simulink model "Simulacion_Realimentacion_del_estado"  (R2017b)
settings: Solver=VariableStepAuto  StartTime=0.0  StopTime=540  RelTol=1e-3
settings Model: Creator=CPOH  LastModifiedBy=CPOH

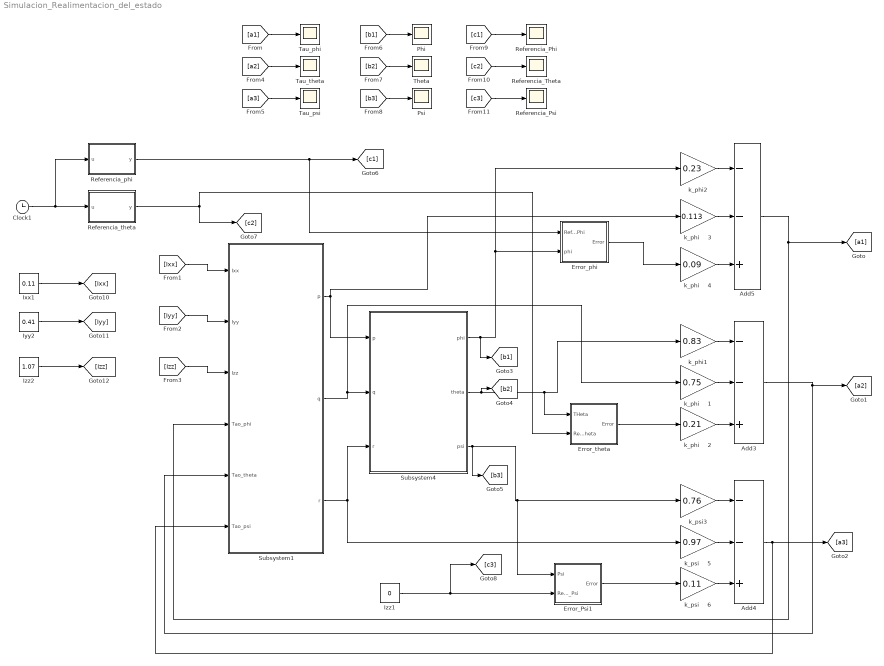
== system Simulacion_Realimentacion_del_estado ==
  Add3 : Sum  Inputs=--+
  Add4 : Sum  Inputs=--+
  Add5 : Sum  Inputs=--+
  Clock1 : Clock
  Error_Psi1 : Subsystem
  Error_phi : Subsystem
  Error_theta : Subsystem
  Ixx1 : Constant  Value=0.11
  Iyy2 : Constant  Value=0.41
  Izz1 : Constant  Value=0
  Izz2 : Constant  Value=1.07
  Phi : Scope
  Psi : Scope
  Referencia_Phi : Scope
  Referencia_Psi : Scope
  Referencia_Theta : Scope
  Referencia_phi : MATLAB Function  TreatAsAtomicUnit=on
  Referencia_theta : MATLAB Function  TreatAsAtomicUnit=on
  Subsystem1 : Subsystem
  Subsystem4 : Subsystem
  Tau_phi : Scope
  Tau_psi : Scope
  Tau_theta : Scope
  Theta : Scope
  k_phi     1 : Gain  Gain=0.75
  k_phi     2 : Gain  Gain=0.21
  k_phi     3 : Gain  Gain=0.113
  k_phi     4 : Gain  Gain=0.09
  k_phi1 : Gain  Gain=0.83
  k_phi2 : Gain  Gain=0.23
  k_psi     5 : Gain  Gain=0.97
  k_psi     6 : Gain  Gain=0.11
  k_psi3 : Gain  Gain=0.76
  wires:
  k_phi     4/1 -> Add5/3
  Subsystem4/2(theta) -> [b2], Error_theta/1(THeta), k_phi1/1
  Iyy2/1 -> [Iyy]
  Clock1/1 -> Referencia_phi/1(u), Referencia_theta/1(u)
  k_phi2/1 -> Add5/1
  Referencia_theta/1(y) -> Error_theta/2(Referencia_theta), [c2]
  Subsystem1/1(p) -> k_phi     3/1, Subsystem4/1(p)
  Subsystem1/3(r) -> Subsystem4/3(r), k_psi     5/1
  [Iyy] -> Subsystem1/2(Iyy)
  k_phi1/1 -> Add3/1
  k_phi     1/1 -> Add3/2
  Ixx1/1 -> [Ixx]
  Izz2/1 -> [Izz]
  Add3/1 -> [a2], Subsystem1/5(Tao_theta)
  [Ixx] -> Subsystem1/1(Ixx)
  k_psi3/1 -> Add4/1
  Error_phi/1(Error) -> k_phi     4/1
  Error_Psi1/1(Error) -> k_psi     6/1
  Error_theta/1(Error) -> k_phi     2/1
  k_psi     5/1 -> Add4/2
  Referencia_phi/1(y) -> [c1], Error_phi/1(Referencia_Phi)
  k_psi     6/1 -> Add4/3
  k_phi     3/1 -> Add5/2
  [Izz] -> Subsystem1/3(Izz)
  Add4/1 -> Subsystem1/6("Tao_psi "), [a3]
  k_phi     2/1 -> Add3/3
  Subsystem4/3(psi) -> Error_Psi1/1(Psi), k_psi3/1, [b3]
  Subsystem1/2(q) -> k_phi     1/1, Subsystem4/2(q)
  Add5/1 -> [a1], Subsystem1/4(Tao_phi)
  Izz1/1 -> [c3], Error_Psi1/2(Referencia_Psi)
  [a1] -> Tau_phi/1
  [a2] -> Tau_theta/1
  [a3] -> Tau_psi/1
  [b1] -> Phi/1
  [b2] -> Theta/1
  [b3] -> Psi/1
  [c1] -> Referencia_Phi/1
  [c2] -> Referencia_Theta/1
  [c3] -> Referencia_Psi/1
  Subsystem4/1(phi) -> [b1], Error_phi/2(phi), k_phi2/1

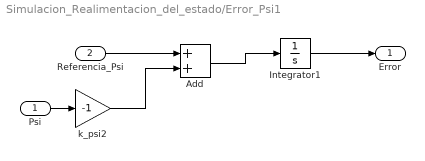
== system Simulacion_Realimentacion_del_estado/Error_Psi1 ==
  Psi : Inport
  Referencia_Psi : Inport  Port=2
  Add : Sum
  Integrator1 : Integrator
  k_psi2 : Gain  Gain=-1
  Error : Outport
  wires:
  Psi/1 -> k_psi2/1
  Referencia_Psi/1 -> Add/1
  Integrator1/1 -> Error/1
  Add/1 -> Integrator1/1
  k_psi2/1 -> Add/2

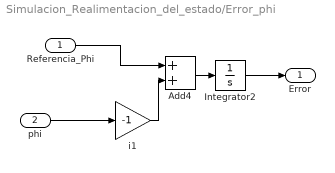
== system Simulacion_Realimentacion_del_estado/Error_phi ==
  Referencia_Phi : Inport
  phi : Inport  Port=2
  Add4 : Sum
  Integrator2 : Integrator
  i1 : Gain  Gain=-1
  Error : Outport
  wires:
  Integrator2/1 -> Error/1
  i1/1 -> Add4/2
  Add4/1 -> Integrator2/1
  Referencia_Phi/1 -> Add4/1
  phi/1 -> i1/1

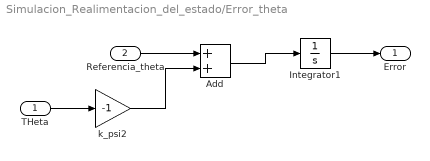
== system Simulacion_Realimentacion_del_estado/Error_theta ==
  THeta : Inport
  Referencia_theta : Inport  Port=2
  Add : Sum
  Integrator1 : Integrator
  k_psi2 : Gain  Gain=-1
  Error : Outport
  wires:
  k_psi2/1 -> Add/2
  Add/1 -> Integrator1/1
  Integrator1/1 -> Error/1
  Referencia_theta/1 -> Add/1
  THeta/1 -> k_psi2/1

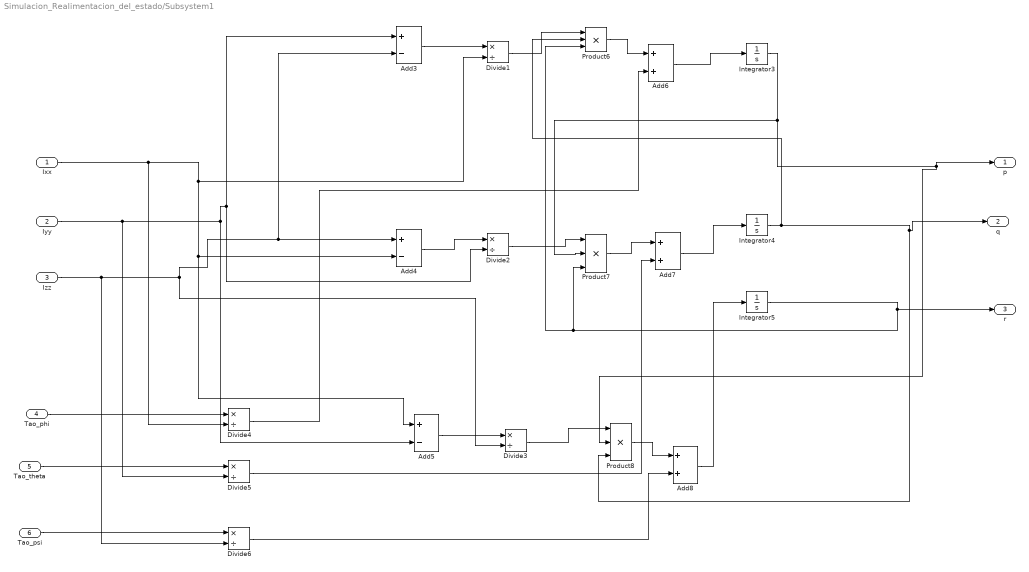
== system Simulacion_Realimentacion_del_estado/Subsystem1 ==
  Ixx : Inport
  Iyy : Inport  Port=2
  Izz : Inport  Port=3
  Tao_phi : Inport  Port=4
  Tao_theta : Inport  Port=5
  "Tao_psi " : Inport  Port=6
  Add3 : Sum  Inputs=+-
  Add4 : Sum  Inputs=+-
  Add5 : Sum  Inputs=+-
  Add6 : Sum
  Add7 : Sum
  Add8 : Sum
  Divide{1..6} (6 alike) : Product  Inputs=*/
  Integrator3 : Integrator
  Integrator4 : Integrator
  Integrator5 : Integrator
  Product6 : Product  Inputs=3
  Product7 : Product  Inputs=3
  Product8 : Product  Inputs=3
  p : Outport
  q : Outport  Port=2
  r : Outport  Port=3
  wires:
  Divide3/1 -> Product8/1
  Divide2/1 -> Product7/1
  Product7/1 -> Add7/1
  Product6/1 -> Add6/1
  Add3/1 -> Divide1/1
  Add4/1 -> Divide2/1
  Divide1/1 -> Product6/1
  Tao_theta/1 -> Divide5/1
  Divide4/1 -> Add6/2
  Ixx/1 -> Divide1/2, Add4/2, Add5/1, Divide4/2
  Izz/1 -> Divide3/2, Add3/2, Add4/1, Divide6/2
  Tao_phi/1 -> Divide4/1
  Divide5/1 -> Add7/2
  "Tao_psi "/1 -> Divide6/1
  Divide6/1 -> Add8/2
  Integrator3/1 -> Product7/2, p/1, Product8/2
  Product8/1 -> Add8/1
  Integrator4/1 -> Product6/2, Product8/3, q/1
  Integrator5/1 -> Product6/3, Product7/3, r/1
  Add5/1 -> Divide3/1
  Add7/1 -> Integrator4/1
  Iyy/1 -> Add5/2, Divide2/2, Add3/1, Divide5/2
  Add6/1 -> Integrator3/1
  Add8/1 -> Integrator5/1

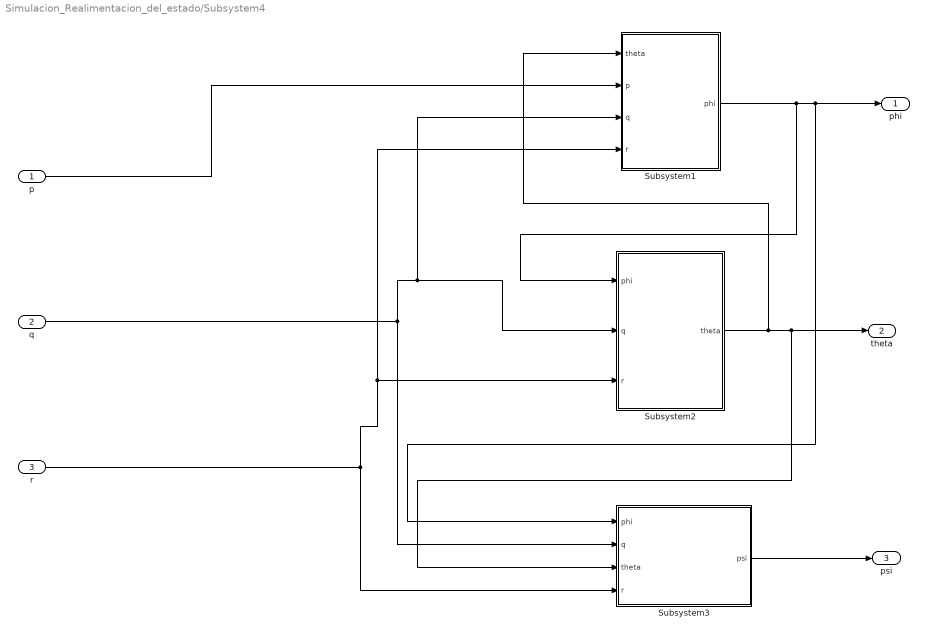
== system Simulacion_Realimentacion_del_estado/Subsystem4 ==
  p : Inport
  q : Inport  Port=2
  r : Inport  Port=3
  Subsystem1 : Subsystem
  Subsystem2 : Subsystem
  Subsystem3 : Subsystem
  phi : Outport
  theta : Outport  Port=2
  psi : Outport  Port=3
  wires:
  Subsystem2/1(theta) -> Subsystem1/1(theta), Subsystem3/3(theta), theta/1
  Subsystem1/1(phi) -> Subsystem2/1(phi), Subsystem3/1(phi), phi/1
  p/1 -> Subsystem1/2(p)
  Subsystem3/1(psi) -> psi/1
  r/1 -> Subsystem3/4(r), Subsystem1/4(r), Subsystem2/3(r)
  q/1 -> Subsystem3/2(q), Subsystem1/3(q), Subsystem2/2(q)

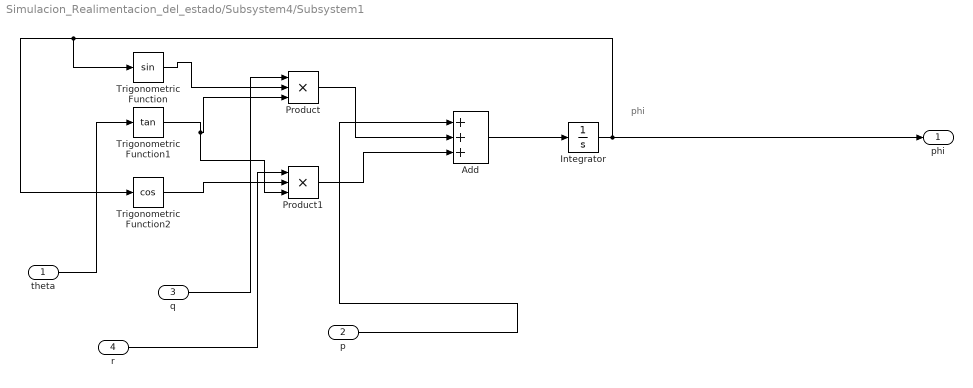
== system Simulacion_Realimentacion_del_estado/Subsystem4/Subsystem1 ==
  note: phi
  theta : Inport
  p : Inport  Port=2
  q : Inport  Port=3
  r : Inport  Port=4
  Add : Sum  Inputs=+++
  Integrator : Integrator
  Product : Product  Inputs=3
  Product1 : Product  Inputs=3
  Trigonometric Function : Trigonometry
  Trigonometric Function1 : Trigonometry  Operator=tan
  Trigonometric Function2 : Trigonometry  Operator=cos
  phi : Outport
  wires:
  p/1 -> Add/1
  q/1 -> Product/1
  r/1 -> Product1/1
  Add/1 -> Integrator/1
  Trigonometric Function1/1 -> Product/3, Product1/3
  Trigonometric Function2/1 -> Product1/2
  Product/1 -> Add/2
  Trigonometric Function/1 -> Product/2
  Integrator/1 -> Trigonometric Function/1, Trigonometric Function2/1, phi/1
  Product1/1 -> Add/3
  theta/1 -> Trigonometric Function1/1

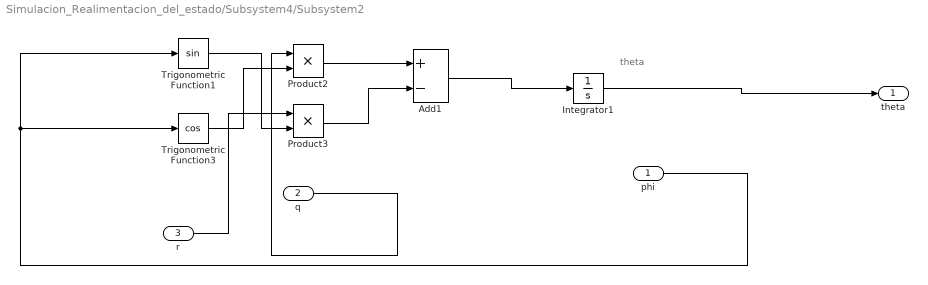
== system Simulacion_Realimentacion_del_estado/Subsystem4/Subsystem2 ==
  note: theta
  phi : Inport
  q : Inport  Port=2
  r : Inport  Port=3
  Add1 : Sum  Inputs=+-
  Integrator1 : Integrator
  Product2 : Product
  Product3 : Product
  Trigonometric Function1 : Trigonometry
  Trigonometric Function3 : Trigonometry  Operator=cos
  theta : Outport
  wires:
  Trigonometric Function3/1 -> Product2/2
  Product2/1 -> Add1/1
  Add1/1 -> Integrator1/1
  Integrator1/1 -> theta/1
  Product3/1 -> Add1/2
  r/1 -> Product3/1
  phi/1 -> Trigonometric Function3/1, Trigonometric Function1/1
  q/1 -> Product2/1
  Trigonometric Function1/1 -> Product3/2

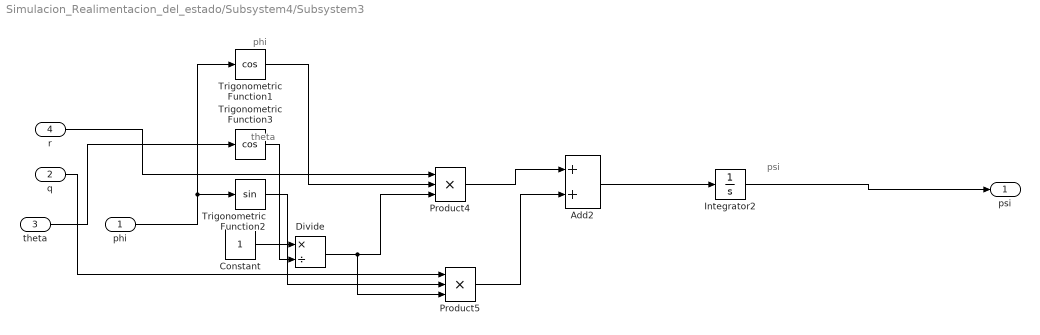
== system Simulacion_Realimentacion_del_estado/Subsystem4/Subsystem3 ==
  note: psi
  note: phi
  note: theta
  phi : Inport
  q : Inport  Port=2
  theta : Inport  Port=3
  r : Inport  Port=4
  Add2 : Sum
  Constant : Constant
  Divide : Product  Inputs=*/
  Integrator2 : Integrator
  Product4 : Product  Inputs=3
  Product5 : Product  Inputs=3
  Trigonometric Function1 : Trigonometry  Operator=cos
  Trigonometric Function2 : Trigonometry
  Trigonometric Function3 : Trigonometry  Operator=cos
  psi : Outport
  wires:
  phi/1 -> Trigonometric Function1/1, Trigonometric Function2/1
  r/1 -> Product4/1
  theta/1 -> Trigonometric Function3/1
  q/1 -> Product5/1
  Constant/1 -> Divide/1
  Trigonometric Function2/1 -> Product5/2
  Product5/1 -> Add2/2
  Add2/1 -> Integrator2/1
  Trigonometric Function1/1 -> Product4/2
  Divide/1 -> Product4/3, Product5/3
  Product4/1 -> Add2/1
  Trigonometric Function3/1 -> Divide/2
  Integrator2/1 -> psi/1

== matlab function Simulacion_Realimentacion_del_estado/Referencia_phi ==
  data: u input; y output
function y = fcn(u)

e=0;
offset=70;
if u>103.8-offset
 e=0.3;   
end

if u>160.8-offset
     e=-0.1;  
end

if u>219.7-offset
     e=0;  
end

if u>280.2-offset
    e=-0.2;
end

if u>339.8-offset
    e=0.3;
end


if u>388.54-offset
    e=0;
end



y = e;

== matlab function Simulacion_Realimentacion_del_estado/Referencia_theta ==
  data: u input; y output
function y = fcn(u)

e=0;
offset=70;
if u>103.8-offset
 e=-0.2;   
end

if u>160.8-offset
     e=0.3;  
end

if u>219.7-offset
     e=0;  
end

if u>280.2-offset
     e=0.3;  
end

if u>339.8-offset
    e=-0.1;
end

if u>388.54-offset
    e=0;
end








y = e;
